simulink model "FusionMODEL_version4"  (R2018a)
settings: Solver=FixedStepAuto  StartTime=0.0  StopTime=SimulationTime  FixedStep=SamplingTime  RelTol=1e-3
values from neighbouring files (symbols this model uses):
  ValidateGRID = true    [SensorFusion_Script0_main.m]
  ValidateLAYOUT = true    [SensorFusion_Script0_main.m]
  VisualizeCLUSTERING = true    [SensorFusion_Script0_main.m]
undefined symbols (not defined in the file or in its folder): ACTIVATE_CAM, ACTIVATE_RAD, CAM1_detTimeStamp, CAM1_MeasNoise, CAM1_objClassID, CAM1_PX, CAM1_PY, CAM1_VX, CAM1_VY, CAM2_detTimeStamp, CAM2_MeasNoise, CAM2_objClassID, CAM2_PX, CAM2_PY, CAM2_VX, CAM2_VY, CAM3_detTimeStamp, CAM3_MeasNoise, CAM3_objClassID, CAM3_PX, CAM3_PY, CAM3_VX, CAM3_VY, CAM4_detTimeStamp, CAM4_MeasNoise, CAM4_objClassID, CAM4_PX, CAM4_PY, CAM4_VX, CAM4_VY, CAM5_detTimeStamp, CAM5_MeasNoise, CAM5_objClassID, CAM5_PX, CAM5_PY, CAM5_VX, CAM5_VY, CAM6_detTimeStamp, CAM6_MeasNoise, CAM6_objClassID, CAM6_PX, CAM6_PY, CAM6_VX, CAM6_VY, CAM7_detTimeStamp, CAM7_MeasNoise, CAM7_objClassID, CAM7_PX, CAM7_PY, CAM7_VX, CAM7_VY, CAM8_detTimeStamp, CAM8_MeasNoise, CAM8_objClassID, CAM8_PX, CAM8_PY, CAM8_VX, CAM8_VY, CAM_nMeas, CAM_TYPE ... (+171)
libraries: simulink_extras x4
(part 8 of 9)

== system FusionMODEL_version4/OBJECT_TRACKER_SENSOR_FUSION/NEAREST_NEIGHBOUR_FOR_CAMERA_MEASUREMENT_GROUPING/NN_MEASUREMENT_GROUPING_WITHIN_EPS/For Iterator Subsystem/NN/PERFORM_NN_CLUSTERING/CHECK_CONDITION ==
  MEAS : Inport
  idx_i : Inport  Port=2
  idx_j : Inport  Port=3
  CLSTR_DATA_INIT : Inport  Port=4
  CLSTR_DATA_PREV : Inport  Port=5
  Bus Selector : BusSelector  OutputSignals=isMeasVisitedFlag
  Bus Selector1 : BusSelector  OutputSignals=MeasArray
  Constant2 : Constant  Value=nn_eps
  LessThanOrEqual1 : RelationalOperator  Operator=<=  OutDataTypeStr=boolean  RndMeth=Simplest
  Logical Operator : Logic  AllPortsSameDT=off  OutDataTypeStr=boolean
  Logical Operator1 : Logic  Operator=NOT  AllPortsSameDT=off  OutDataTypeStr=boolean
  Selector1 : Selector  NumberOfDimensions=2  InputPortWidth=3  IndexOptions=Select all,Index vector (port)  Indices=[1 3],1  OutputSizes=1,1
  Selector2 : Selector  NumberOfDimensions=2  InputPortWidth=3  IndexOptions=Select all,Index vector (port)  Indices=[1 3],1  OutputSizes=1,1
  Selector3 : Selector  NumberOfDimensions=2  InputPortWidth=3  IndexOptions=Select all,Index vector (port)  Indices=[1 3],1  OutputSizes=1,1
  Sqrt : Sqrt  SaturateOnIntegerOverflow=on
  Square : Math  Operator=square  SaturateOnIntegerOverflow=on
  Subtract : Sum  Inputs=+-
  Sum of Elements : Sum  Inputs=+
  Switch6 : Switch  Criteria=u2 > Threshold  Threshold=int32(1)
  Unit Delay : UnitDelay  InitialCondition=CLSTR_SNSR_DELAY_INIT  SampleTime=-1
  isMember : Outport
  CLSTR_DATA : Outport  Port=2
  wires:
  LessThanOrEqual1/1 -> Logical Operator/1
  Bus Selector/1 -> Selector1/1  "<isMeasVisitedFlag>"
  Logical Operator1/1 -> Logical Operator/2
  [x_i] -> Selector2/2
  Bus Selector1/1 -> Selector2/1, Selector3/1  "<MeasArray>"
  Sqrt/1 -> LessThanOrEqual1/1
  idx_i/1 -> [x_i]
  Selector1/1 -> Logical Operator1/1
  idx_j/1 -> [y_j]
  [y_j] -> Selector3/2
  Selector3/1 -> Subtract/2
  Constant2/1 -> LessThanOrEqual1/2
  Selector2/1 -> Subtract/1
  Logical Operator/1 -> isMember/1
  [y_j] -> Selector1/2
  Subtract/1 -> Square/1
  MEAS/1 -> Bus Selector1/1
  Square/1 -> Sum of Elements/1
  Sum of Elements/1 -> Sqrt/1
  [y_j] -> Switch6/2
  CLSTR_DATA_INIT/1 -> Switch6/3
  Switch6/1 -> Bus Selector/1, CLSTR_DATA/1
  CLSTR_DATA_PREV/1 -> Unit Delay/1
  Unit Delay/1 -> Switch6/1

== system FusionMODEL_version4/OBJECT_TRACKER_SENSOR_FUSION/NEAREST_NEIGHBOUR_FOR_CAMERA_MEASUREMENT_GROUPING/NN_MEASUREMENT_GROUPING_WITHIN_EPS/For Iterator Subsystem/NN/PERFORM_NN_CLUSTERING/SET_DATA ==
  isClusterMember : Inport
  CLSTR_DATA : Inport  Port=2
  idx_j : Inport  Port=3
  GET_DATA_FROM_BUS : Subsystem
  SET_CLUSTER_DATA_TO_BUS : Subsystem
  UPDATE_CLUSTER_DATA1 : Subsystem
  CLSTR_DATA_UPD : Outport
  wires:
  SET_CLUSTER_DATA_TO_BUS/1(CLSTR_DATA_UPD) -> CLSTR_DATA_UPD/1
  isClusterMember/1 -> UPDATE_CLUSTER_DATA1/1(FLAG)
  idx_j/1 -> UPDATE_CLUSTER_DATA1/2(idx_j)
  GET_DATA_FROM_BUS/1(<ClusterSizes>) -> UPDATE_CLUSTER_DATA1/3(ClusterSizes)
  GET_DATA_FROM_BUS/2(<ClusterToMeasAssignment>) -> UPDATE_CLUSTER_DATA1/4(Clstr2MeasAssign)
  GET_DATA_FROM_BUS/3(<isMeasVisitedFlag>) -> UPDATE_CLUSTER_DATA1/5(MeasIsVisited)
  GET_DATA_FROM_BUS/4(<nClusters>) -> UPDATE_CLUSTER_DATA1/6(nClusters)
  GET_DATA_FROM_BUS/5(<ClusterMember>) -> UPDATE_CLUSTER_DATA1/7(ClstrMem)
  CLSTR_DATA/1 -> SET_CLUSTER_DATA_TO_BUS/5(CLSTR_DATA), GET_DATA_FROM_BUS/1(CLSTR_DATA)
  UPDATE_CLUSTER_DATA1/1(isVisited) -> SET_CLUSTER_DATA_TO_BUS/1(isMeasVisitedFlag)
  UPDATE_CLUSTER_DATA1/2(ClstrSize) -> SET_CLUSTER_DATA_TO_BUS/2(ClusterSizes)
  UPDATE_CLUSTER_DATA1/3(ClstrAssignment) -> SET_CLUSTER_DATA_TO_BUS/3(ClusterToMeasAssignment)
  UPDATE_CLUSTER_DATA1/4(ClstrMember) -> SET_CLUSTER_DATA_TO_BUS/4(ClusterMember)

== system FusionMODEL_version4/OBJECT_TRACKER_SENSOR_FUSION/SENSOR_LAYOUT_AND_CHRACTERIZATION/PRE_COMPUTE_SENSOR_FOV_GRID/COMPUTE_CAMERA_SNSR_GRID/ComputeCoverageANDConfidence/Compute_Cell_X_and_Y_index/Compute_Cell_X_Y_Center_Coordinate ==
  Cell_id : Inport
  xRes : Inport  Port=2
  xRear : Inport  Port=3
  Cy : Inport  Port=4
  yRes : Inport  Port=5
  yLeft : Inport  Port=6
  Add : Sum  Inputs=+++
  Add1 : Sum  Inputs=+++
  Constant : Constant  Value=single(0.5)
  Divide : Product  Inputs=*/
  Divide1 : Product  Inputs=/*
  Divide2 : Product  Inputs=*/
  Floor : Rounding
  Floor1 : Rounding
  Floor2 : Rounding
  Multiply : Product
  Multiply1 : Product
  Multiply2 : Product
  Subtract : Sum  Inputs=+-
  CellCenterCoordX : Outport
  CellCenterCoordY : Outport  Port=2
  wires:
  Cell_id/1 -> Subtract/1, Divide/1
  Cy/1 -> Multiply/2, Divide/2
  Divide/1 -> Floor/1
  Floor/1 -> [Grid_x_index], Multiply/1
  Multiply/1 -> Subtract/2
  yLeft/1 -> Divide2/1
  yRes/1 -> Multiply1/2, Divide2/2
  Divide1/1 -> Floor1/1
  Divide2/1 -> Floor2/1
  Subtract/1 -> [Grid_y_index]
  Floor1/1 -> Add/2
  [Grid_x_index] -> Add/1
  Constant/1 -> Add1/1, Add/3
  Floor2/1 -> Add1/2
  [Grid_y_index] -> Add1/3
  Add1/1 -> Multiply1/1
  Multiply1/1 -> CellCenterCoordY/1
  xRear/1 -> Divide1/2
  xRes/1 -> Multiply2/1, Divide1/1
  Add/1 -> Multiply2/2
  Multiply2/1 -> CellCenterCoordX/1

== system FusionMODEL_version4/OBJECT_TRACKER_SENSOR_FUSION/SENSOR_LAYOUT_AND_CHRACTERIZATION/PRE_COMPUTE_SENSOR_FOV_GRID/COMPUTE_CAMERA_SNSR_GRID/ComputeCoverageANDConfidence/Compute_Cell_X_and_Y_index/Compute_FOV_Overlap_with_Cell_and_Region_Confidence ==
  Cell_xSnsrCoord : Inport
  Cell_ySnsrCoord : Inport  Port=2
  SnsrIntrinsic : Inport  Port=3
  If : If  ElseIfExpressions=u1 <= 0  ShowElse=off
  If Action Subsystem : Subsystem  TreatAsAtomicUnit=on
  If Action Subsystem2 : Subsystem  TreatAsAtomicUnit=on
  Merge : Merge
  Merge1 : Merge
  RegionConfidence : Outport
  FOVOverlap : Outport  Port=2
  wires:
  If/1 -> If Action Subsystem/Action
  If/2 -> If Action Subsystem2/Action
  If Action Subsystem/1(RegionConfidence) -> [Confi1]
  If Action Subsystem2/1(RegionConfidence) -> [Confi2]
  [Confi1] -> Merge/1
  [Confi2] -> Merge/2
  If Action Subsystem/2(fovOverlap) -> [Overlap1]
  If Action Subsystem2/2(fovOverlap) -> [Overlap2]
  [Overlap1] -> Merge1/1
  [Overlap2] -> Merge1/2
  Cell_xSnsrCoord/1 -> [Cell_xCoord]
  Cell_ySnsrCoord/1 -> [Cell_yCoord]
  [Cell_xCoord] -> If/1
  [Cell_yCoord] -> If Action Subsystem/2(Cell_ySnsrCoord)
  [Cell_xCoord] -> If Action Subsystem/1(Cell_xSnsrCoord)
  SnsrIntrinsic/1 -> [SnsrIntrinsic]
  [SnsrIntrinsic] -> If Action Subsystem/3(SnsrIntrinsic)
  Merge1/1 -> FOVOverlap/1
  Merge/1 -> RegionConfidence/1

== system FusionMODEL_version4/OBJECT_TRACKER_SENSOR_FUSION/SENSOR_LAYOUT_AND_CHRACTERIZATION/PRE_COMPUTE_SENSOR_FOV_GRID/COMPUTE_CAMERA_SNSR_GRID/ComputeCoverageANDConfidence/Compute_Cell_X_and_Y_index/GET_DATA ==
  GridID_vector : Inport
  index : Inport  Port=2
  GridParam : Inport  Port=3
  Bus Selector : BusSelector  OutputSignals=xGridParameters,yGridParameters
  Bus Selector1 : BusSelector  OutputSignals=nGridCellsLat,yRes,yLeft
  Bus Selector2 : BusSelector  OutputSignals=xRes,xRear
  Selector : Selector  NumberOfDimensions=2  InputPortWidth=3  IndexOptions=Select all,Index vector (port)  Indices=[1 3],1  OutputSizes=1,1
  CellID : Outport
  <xRes> : Outport  Port=2
  <xRear> : Outport  Port=3
  <nGridCellsLat> : Outport  Port=4
  <yRes> : Outport  Port=5
  <yLeft> : Outport  Port=6
  wires:
  Bus Selector/2 -> Bus Selector1/1  "<yGridParameters>"
  Bus Selector/1 -> Bus Selector2/1  "<xGridParameters>"
  Bus Selector2/2 -> <xRear>/1  "<xRear>"
  GridParam/1 -> Bus Selector/1
  GridID_vector/1 -> Selector/1
  Selector/1 -> CellID/1
  Bus Selector1/2 -> <yRes>/1  "<yRes>"
  index/1 -> Selector/2
  Bus Selector2/1 -> <xRes>/1  "<xRes>"
  Bus Selector1/1 -> <nGridCellsLat>/1  "<nGridCellsLat>"
  Bus Selector1/3 -> <yLeft>/1  "<yLeft>"

== system FusionMODEL_version4/OBJECT_TRACKER_SENSOR_FUSION/SENSOR_LAYOUT_AND_CHRACTERIZATION/PRE_COMPUTE_SENSOR_FOV_GRID/COMPUTE_CAMERA_SNSR_GRID/ComputeCoverageANDConfidence/Compute_Cell_X_and_Y_index/Transform_Cell_Coordinate_Vehicle_Frame_To_Sensor_Frame ==
  Cell_xCoord : Inport
  Cell_y_Coord : Inport  Port=2
  SensorExtrinsic : Inport  Port=3
  Bus Selector : BusSelector  OutputSignals=RotMat2D,TranslationVec
  Matrix Multiply : Product  Multiplication=Matrix(*)
  Mux : Mux  Inputs=2
  Reshape : Reshape  OutputDimensionality=Column vector (2-D)
  Selector : Selector  NumberOfDimensions=2  InputPortWidth=3  IndexOptions=Index vector (dialog),Select all  Indices=1,1  OutputSizes=1,1
  Selector1 : Selector  NumberOfDimensions=2  InputPortWidth=3  IndexOptions=Index vector (dialog),Select all  Indices=2,1  OutputSizes=1,1
  Subtract : Sum  Inputs=-+
  Transpose : Math  Operator=transpose  SaturateOnIntegerOverflow=on
  Cell_xSnsrCoord : Outport
  Cell_ySnsrCoord : Outport  Port=2
  wires:
  SensorExtrinsic/1 -> Bus Selector/1
  Cell_xCoord/1 -> Mux/1
  Cell_y_Coord/1 -> Mux/2
  Mux/1 -> Reshape/1
  Bus Selector/1 -> Transpose/1  "<RotMat2D>"
  Bus Selector/2 -> Subtract/1  "<TranslationVec>"
  Reshape/1 -> Subtract/2
  Transpose/1 -> Matrix Multiply/1
  Subtract/1 -> Matrix Multiply/2
  Matrix Multiply/1 -> Selector1/1, Selector/1
  Selector/1 -> Cell_xSnsrCoord/1
  Selector1/1 -> Cell_ySnsrCoord/1

== system FusionMODEL_version4/OBJECT_TRACKER_SENSOR_FUSION/SENSOR_LAYOUT_AND_CHRACTERIZATION/PRE_COMPUTE_SENSOR_FOV_GRID/COMPUTE_RADAR_SNSR_GRID/ComputeCoverageANDConfidence/Compute_Cell_X_and_Y_index/Compute_Cell_X_Y_Center_Coordinate ==
  Cell_id : Inport
  xRes : Inport  Port=2
  xRear : Inport  Port=3
  Cy : Inport  Port=4
  yRes : Inport  Port=5
  yLeft : Inport  Port=6
  Add : Sum  Inputs=+++
  Add1 : Sum  Inputs=+++
  Constant : Constant  Value=single(0.5)
  Divide : Product  Inputs=*/
  Divide1 : Product  Inputs=/*
  Divide2 : Product  Inputs=*/
  Floor : Rounding
  Floor1 : Rounding
  Floor2 : Rounding
  Multiply : Product
  Multiply1 : Product
  Multiply2 : Product
  Subtract : Sum  Inputs=+-
  CellCenterCoordX : Outport
  CellCenterCoordY : Outport  Port=2
  wires:
  Cell_id/1 -> Subtract/1, Divide/1
  Cy/1 -> Multiply/2, Divide/2
  Divide/1 -> Floor/1
  Floor/1 -> [Grid_x_index], Multiply/1
  Multiply/1 -> Subtract/2
  yLeft/1 -> Divide2/1
  yRes/1 -> Multiply1/2, Divide2/2
  Divide1/1 -> Floor1/1
  Divide2/1 -> Floor2/1
  Subtract/1 -> [Grid_y_index]
  Floor1/1 -> Add/2
  [Grid_x_index] -> Add/1
  Constant/1 -> Add1/1, Add/3
  Floor2/1 -> Add1/2
  [Grid_y_index] -> Add1/3
  Add1/1 -> Multiply1/1
  Multiply1/1 -> CellCenterCoordY/1
  xRear/1 -> Divide1/2
  xRes/1 -> Multiply2/1, Divide1/1
  Add/1 -> Multiply2/2
  Multiply2/1 -> CellCenterCoordX/1

== system FusionMODEL_version4/OBJECT_TRACKER_SENSOR_FUSION/SENSOR_LAYOUT_AND_CHRACTERIZATION/PRE_COMPUTE_SENSOR_FOV_GRID/COMPUTE_RADAR_SNSR_GRID/ComputeCoverageANDConfidence/Compute_Cell_X_and_Y_index/Compute_FOV_Overlap_with_Cell_and_Region_Confidence ==
  Cell_xSnsrCoord : Inport
  Cell_ySnsrCoord : Inport  Port=2
  SnsrIntrinsic : Inport  Port=3
  If : If  ElseIfExpressions=u1 <= 0  ShowElse=off
  If Action Subsystem : Subsystem  TreatAsAtomicUnit=on
  If Action Subsystem2 : Subsystem  TreatAsAtomicUnit=on
  Merge : Merge
  Merge1 : Merge
  RegionConfidence : Outport
  FOVOverlap : Outport  Port=2
  wires:
  If/1 -> If Action Subsystem/Action
  If/2 -> If Action Subsystem2/Action
  If Action Subsystem/1(RegionConfidence) -> [Confi1]
  If Action Subsystem2/1(RegionConfidence) -> [Confi2]
  [Confi1] -> Merge/1
  [Confi2] -> Merge/2
  If Action Subsystem/2(fovOverlap) -> [Overlap1]
  If Action Subsystem2/2(fovOverlap) -> [Overlap2]
  [Overlap1] -> Merge1/1
  [Overlap2] -> Merge1/2
  Cell_xSnsrCoord/1 -> [Cell_xCoord]
  Cell_ySnsrCoord/1 -> [Cell_yCoord]
  [Cell_xCoord] -> If/1
  [Cell_yCoord] -> If Action Subsystem/2(Cell_ySnsrCoord)
  [Cell_xCoord] -> If Action Subsystem/1(Cell_xSnsrCoord)
  SnsrIntrinsic/1 -> [SnsrIntrinsic]
  [SnsrIntrinsic] -> If Action Subsystem/3(SnsrIntrinsic)
  Merge1/1 -> FOVOverlap/1
  Merge/1 -> RegionConfidence/1

== system FusionMODEL_version4/OBJECT_TRACKER_SENSOR_FUSION/SENSOR_LAYOUT_AND_CHRACTERIZATION/PRE_COMPUTE_SENSOR_FOV_GRID/COMPUTE_RADAR_SNSR_GRID/ComputeCoverageANDConfidence/Compute_Cell_X_and_Y_index/GET_DATA ==
  GridID_vector : Inport
  index : Inport  Port=2
  GridParam : Inport  Port=3
  Bus Selector : BusSelector  OutputSignals=xGridParameters,yGridParameters
  Bus Selector1 : BusSelector  OutputSignals=nGridCellsLat,yRes,yLeft
  Bus Selector2 : BusSelector  OutputSignals=xRes,xRear
  Selector : Selector  NumberOfDimensions=2  InputPortWidth=3  IndexOptions=Select all,Index vector (port)  Indices=[1 3],1  OutputSizes=1,1
  CellID : Outport
  <xRes> : Outport  Port=2
  <xRear> : Outport  Port=3
  <nGridCellsLat> : Outport  Port=4
  <yRes> : Outport  Port=5
  <yLeft> : Outport  Port=6
  wires:
  Bus Selector/2 -> Bus Selector1/1  "<yGridParameters>"
  Bus Selector/1 -> Bus Selector2/1  "<xGridParameters>"
  Bus Selector2/2 -> <xRear>/1  "<xRear>"
  GridParam/1 -> Bus Selector/1
  GridID_vector/1 -> Selector/1
  Selector/1 -> CellID/1
  Bus Selector1/2 -> <yRes>/1  "<yRes>"
  index/1 -> Selector/2
  Bus Selector2/1 -> <xRes>/1  "<xRes>"
  Bus Selector1/1 -> <nGridCellsLat>/1  "<nGridCellsLat>"
  Bus Selector1/3 -> <yLeft>/1  "<yLeft>"

== system FusionMODEL_version4/OBJECT_TRACKER_SENSOR_FUSION/SENSOR_LAYOUT_AND_CHRACTERIZATION/PRE_COMPUTE_SENSOR_FOV_GRID/COMPUTE_RADAR_SNSR_GRID/ComputeCoverageANDConfidence/Compute_Cell_X_and_Y_index/Transform_Cell_Coordinate_Vehicle_Frame_To_Sensor_Frame ==
  Cell_xCoord : Inport
  Cell_y_Coord : Inport  Port=2
  SensorExtrinsic : Inport  Port=3
  Bus Selector : BusSelector  OutputSignals=RotMat2D,TranslationVec
  Matrix Multiply : Product  Multiplication=Matrix(*)
  Mux : Mux  Inputs=2
  Reshape : Reshape  OutputDimensionality=Column vector (2-D)
  Selector : Selector  NumberOfDimensions=2  InputPortWidth=3  IndexOptions=Index vector (dialog),Select all  Indices=1,1  OutputSizes=1,1
  Selector1 : Selector  NumberOfDimensions=2  InputPortWidth=3  IndexOptions=Index vector (dialog),Select all  Indices=2,1  OutputSizes=1,1
  Subtract : Sum  Inputs=-+
  Transpose : Math  Operator=transpose  SaturateOnIntegerOverflow=on
  Cell_xSnsrCoord : Outport
  Cell_ySnsrCoord : Outport  Port=2
  wires:
  SensorExtrinsic/1 -> Bus Selector/1
  Cell_xCoord/1 -> Mux/1
  Cell_y_Coord/1 -> Mux/2
  Mux/1 -> Reshape/1
  Bus Selector/1 -> Transpose/1  "<RotMat2D>"
  Bus Selector/2 -> Subtract/1  "<TranslationVec>"
  Reshape/1 -> Subtract/2
  Transpose/1 -> Matrix Multiply/1
  Subtract/1 -> Matrix Multiply/2
  Matrix Multiply/1 -> Selector1/1, Selector/1
  Selector/1 -> Cell_xSnsrCoord/1
  Selector1/1 -> Cell_ySnsrCoord/1

== system FusionMODEL_version4/OBJECT_TRACKER_SENSOR_FUSION/SENSOR_LAYOUT_AND_CHRACTERIZATION/SET_SENSOR_CALLIBRATION_PARAMETER/SET_CAMERA_SENSOR_PARAM/SET_CAMERA_EXTRINSIC_PARAM/SET_CAMERA_EXTRINSIC_PARAM/CreateRotationMatTranslationVector ==
  yawInstall : Inport
  xMount : Inport  Port=2
  yMount : Inport  Port=3
  Cos : Trigonometry  Operator=cos
  Cos2 : Trigonometry
  Degrees to Radians : simulink_extras/Transformations/Degrees to Radians
  Gain1 : Gain  Gain=-1
  Gain2 : Gain  Gain=ROT_CONVENTION
  Mux : Mux
  Mux1 : Mux  Inputs=2
  Reshape : Reshape  OutputDimensionality=Customize  OutputDimensions=[2 2]
  Reshape1 : Reshape  OutputDimensionality=Column vector (2-D)  OutputDimensions=[2 2]
  RotMatrx : Outport
  TranslationVector : Outport  Port=2
  wires:
  Cos/1 -> [cos_theta], Mux/1
  [cos_theta] -> Mux/4
  Reshape/1 -> RotMatrx/1
  Degrees to Radians/1 -> Cos2/1, Cos/1
  Mux/1 -> Reshape/1
  Cos2/1 -> Mux/2, Gain1/1
  xMount/1 -> Mux1/1
  yMount/1 -> Mux1/2
  Mux1/1 -> Reshape1/1
  Reshape1/1 -> TranslationVector/1
  Gain1/1 -> Mux/3
  yawInstall/1 -> Gain2/1
  Gain2/1 -> Degrees to Radians/1

== system FusionMODEL_version4/OBJECT_TRACKER_SENSOR_FUSION/SENSOR_LAYOUT_AND_CHRACTERIZATION/SET_SENSOR_CALLIBRATION_PARAMETER/SET_RADAR_SENSOR_PARAM/SET_RADAR_EXTRINSIC_PARAM/SET_RADAR_EXTRINSIC_PARAM/CREATE_ROTATION_MATRIX_TRANSLATION_VECTOR ==
  yawInstall : Inport
  xMount : Inport  Port=2
  yMount : Inport  Port=3
  Cos : Trigonometry  Operator=cos
  Cos2 : Trigonometry
  Degrees to Radians : simulink_extras/Transformations/Degrees to Radians
  Gain1 : Gain  Gain=-1
  Gain2 : Gain  Gain=ROT_CONVENTION
  Mux : Mux
  Mux1 : Mux  Inputs=2
  Reshape : Reshape  OutputDimensionality=Customize  OutputDimensions=[2 2]
  Reshape1 : Reshape  OutputDimensionality=Column vector (2-D)  OutputDimensions=[2 2]
  RotMatrx : Outport
  TranslationVector : Outport  Port=2
  wires:
  Cos/1 -> [cos_theta], Mux/1
  [cos_theta] -> Mux/4
  Reshape/1 -> RotMatrx/1
  Degrees to Radians/1 -> Cos2/1, Cos/1
  Mux/1 -> Reshape/1
  Cos2/1 -> Mux/2, Gain1/1
  xMount/1 -> Mux1/1
  yMount/1 -> Mux1/2
  Mux1/1 -> Reshape1/1
  Reshape1/1 -> TranslationVector/1
  Gain1/1 -> Mux/3
  yawInstall/1 -> Gain2/1
  Gain2/1 -> Degrees to Radians/1

== system FusionMODEL_version4/OBJECT_TRACKER_SENSOR_FUSION/SIMPLIFIED_DBSCAN_FOR_RADAR_MEASUREMENT_GROUPING/DBSCAN_MEASUREMENT_GROUPING/FORM_CLUSTER/DBSCAN/DBSCAN_PROPAGATE_AND_EXPAND_CLUSTER/CHECK_CONDITION ==
  memberIdx : Inport
  CLSTR_DATA_INIT : Inport  Port=2
  CLSTR_DATA_PREV : Inport  Port=3
  Bus Selector : BusSelector  OutputSignals=ClusterMember
  Constant : Constant  Value=uint16(0)
  NotEqual : RelationalOperator  Operator=~=  OutDataTypeStr=boolean  RndMeth=Simplest
  Selector : Selector  NumberOfDimensions=2  InputPortWidth=3  IndexOptions=Select all,Index vector (port)  Indices=[1 3],1  OutputSizes=1,1
  Switch6 : Switch  Criteria=u2 > Threshold  Threshold=int32(1)
  Unit Delay : UnitDelay  InitialCondition=CLSTR_SNSR_DELAY_INIT  SampleTime=-1
  isMember : Outport
  MeasIndex : Outport  Port=2
  CLSTR_DATA : Outport  Port=3
  wires:
  Switch6/1 -> CLSTR_DATA/1, Bus Selector/1
  Bus Selector/1 -> Selector/1  "<ClusterMember>"
  memberIdx/1 -> [idx_i], Selector/2
  Selector/1 -> MeasIndex/1, NotEqual/1
  Constant/1 -> NotEqual/2
  NotEqual/1 -> isMember/1
  CLSTR_DATA_INIT/1 -> Switch6/3
  [idx_i] -> Switch6/2
  CLSTR_DATA_PREV/1 -> Unit Delay/1
  Unit Delay/1 -> Switch6/1

== system FusionMODEL_version4/OBJECT_TRACKER_SENSOR_FUSION/SIMPLIFIED_DBSCAN_FOR_RADAR_MEASUREMENT_GROUPING/DBSCAN_MEASUREMENT_GROUPING/FORM_CLUSTER/DBSCAN/DBSCAN_PROPAGATE_AND_EXPAND_CLUSTER/DO_NOT_EXPAND_CLUSTER ==
  CLSTR_DATA : Inport
  Action Port : ActionPort  ActionType=then
  CLSTR_DATA_NO_UPD : Outport
  wires:
  CLSTR_DATA/1 -> CLSTR_DATA_NO_UPD/1

== system FusionMODEL_version4/OBJECT_TRACKER_SENSOR_FUSION/SIMPLIFIED_DBSCAN_FOR_RADAR_MEASUREMENT_GROUPING/DBSCAN_MEASUREMENT_GROUPING/FORM_CLUSTER/DBSCAN/DBSCAN_PROPAGATE_AND_EXPAND_CLUSTER/EXPAND_CLUSTER ==
  CLSTR_DATA : Inport
  nMeas : Inport  Port=2
  idx_i : Inport  Port=3
  measArray : Inport  Port=4
  Action Port : ActionPort  ActionType=else
  CLUSTER_EXPANSION : Subsystem  TreatAsAtomicUnit=on
  CLSTR_DATA_UPD : Outport
  wires:
  CLSTR_DATA/1 -> CLUSTER_EXPANSION/3(CLSTR_DATA)
  idx_i/1 -> CLUSTER_EXPANSION/4(idx_i)
  nMeas/1 -> CLUSTER_EXPANSION/1(nMeas)
  measArray/1 -> CLUSTER_EXPANSION/2(measArray)
  CLUSTER_EXPANSION/1(CLSTR_DATA_UPD) -> CLSTR_DATA_UPD/1

== system FusionMODEL_version4/OBJECT_TRACKER_SENSOR_FUSION/SIMPLIFIED_DBSCAN_FOR_RADAR_MEASUREMENT_GROUPING/DBSCAN_MEASUREMENT_GROUPING/FORM_CLUSTER/DBSCAN/DBSCAN_PROPAGATE_AND_EXPAND_CLUSTER/MERGE_SIGNALS ==
  CLSTR_NO_UPD : Inport
  CLSTR_UPD : Inport  Port=2
  Merge1 : Merge
  CLSTR_DATA : Outport
  wires:
  CLSTR_NO_UPD/1 -> Merge1/1
  Merge1/1 -> CLSTR_DATA/1
  CLSTR_UPD/1 -> Merge1/2

== system FusionMODEL_version4/OBJECT_TRACKER_SENSOR_FUSION/SPATIAL_ALLIGNMENT/CAMERA_MEASUREMENTS_SPATIAL_ALLIGNMENT/For Iterator Subsystem/For Iterator Subsystem/CoordinateTransformation1/InfoExtractor ==
  In1 : Inport
  In2 : Inport  Port=2
  Bus Selector : BusSelector  OutputSignals=px,py,vx,vy,NoiseCovarience
  Bus Selector1 : BusSelector  OutputSignals=RotMat2D,TranslationVec
  <px> : Outport
  <py> : Outport  Port=2
  <vx> : Outport  Port=3
  <vy> : Outport  Port=4
  RotMat2D : Outport  Port=5
  TransVec2D : Outport  Port=6
  MeasNoiseCov : Outport  Port=7
  wires:
  Bus Selector/4 -> <vy>/1  "<vy>"
  Bus Selector/2 -> <py>/1  "<py>"
  In1/1 -> Bus Selector/1
  Bus Selector1/1 -> RotMat2D/1  "<RotMat2D>"
  Bus Selector/3 -> <vx>/1  "<vx>"
  Bus Selector1/2 -> TransVec2D/1  "<TranslationVec>"
  Bus Selector/1 -> <px>/1  "<px>"
  In2/1 -> Bus Selector1/1
  Bus Selector/5 -> MeasNoiseCov/1  "<NoiseCovarience>"

== system FusionMODEL_version4/OBJECT_TRACKER_SENSOR_FUSION/SPATIAL_ALLIGNMENT/CAMERA_MEASUREMENTS_SPATIAL_ALLIGNMENT/For Iterator Subsystem/For Iterator Subsystem/CoordinateTransformation1/Meas_Noise_Cov_Transformation ==
  RotMatrix : Inport
  MeasCovarience : Inport  Port=2
  Assignment : Assignment  NumberOfDimensions=2  DiagnosticForDimensions=Warning  IndexOptions=Index vector (dialog),Index vector (dialog)  Indices=[1 2],[1 2]  OutputSizes=1,1
  Assignment1 : Assignment  NumberOfDimensions=2  DiagnosticForDimensions=Warning  IndexOptions=Index vector (dialog),Index vector (dialog)  Indices=[3 4],[3 4]  OutputSizes=1,1
  Matrix Multiply : Product  Inputs=3  Multiplication=Matrix(*)
  Matrix Multiply1 : Product  Inputs=3  Multiplication=Matrix(*)
  Selector : Selector  NumberOfDimensions=2  InputPortWidth=3  IndexOptions=Index vector (dialog),Index vector (dialog)  Indices=[1 2],[1 2]  OutputSizes=1,1
  Selector1 : Selector  NumberOfDimensions=2  InputPortWidth=3  IndexOptions=Index vector (dialog),Index vector (dialog)  Indices=[3 4],[3 4]  OutputSizes=1,1
  Transpose : Math  Operator=transpose  SaturateOnIntegerOverflow=on
  Transpose1 : Math  Operator=transpose  SaturateOnIntegerOverflow=on
  MeasCovTransformed : Outport
  wires:
  Matrix Multiply/1 -> Assignment/2
  [RotationMat] -> Transpose1/1
  Matrix Multiply1/1 -> Assignment1/2
  RotMatrix/1 -> [RotationMat], Matrix Multiply/1
  [NoiseCov] -> Assignment/1
  Transpose1/1 -> Matrix Multiply1/3
  Selector1/1 -> Matrix Multiply1/2
  Assignment/1 -> Assignment1/1
  Selector/1 -> Matrix Multiply/2
  [RotationMat] -> Matrix Multiply1/1, Transpose/1
  Transpose/1 -> Matrix Multiply/3
  MeasCovarience/1 -> Selector1/1, [NoiseCov], Selector/1
  Assignment1/1 -> MeasCovTransformed/1

== system FusionMODEL_version4/OBJECT_TRACKER_SENSOR_FUSION/SPATIAL_ALLIGNMENT/CAMERA_MEASUREMENTS_SPATIAL_ALLIGNMENT/For Iterator Subsystem/For Iterator Subsystem/CoordinateTransformation1/Position_Transformation ==
  Px : Inport
  Py : Inport  Port=2
  RotationMat : Inport  Port=3
  TranslationVector : Inport  Port=4
  Add : Sum
  Matrix Multiply : Product  Multiplication=Matrix(*)
  Mux : Mux  Inputs=2
  Reshape : Reshape  OutputDimensionality=Column vector (2-D)
  Selector : Selector  InputPortWidth=2  IndexOptions=Index vector (dialog)  Indices=1  OutputSizes=1
  Selector1 : Selector  InputPortWidth=2  IndexOptions=Index vector (dialog)  Indices=2  OutputSizes=1
  PosXcts : Outport
  PosYcts : Outport  Port=2
  wires:
  Reshape/1 -> Matrix Multiply/2
  Px/1 -> Mux/1
  Py/1 -> Mux/2
  Mux/1 -> Reshape/1
  RotationMat/1 -> Matrix Multiply/1
  Matrix Multiply/1 -> Add/1
  TranslationVector/1 -> Add/2
  Add/1 -> Selector1/1, Selector/1
  Selector/1 -> PosXcts/1
  Selector1/1 -> PosYcts/1

== system FusionMODEL_version4/OBJECT_TRACKER_SENSOR_FUSION/SPATIAL_ALLIGNMENT/CAMERA_MEASUREMENTS_SPATIAL_ALLIGNMENT/For Iterator Subsystem/For Iterator Subsystem/CoordinateTransformation1/Subsystem ==
  pxCTS : Inport
  pyCTS : Inport  Port=2
  vxCTS : Inport  Port=3
  vyCTS : Inport  Port=4
  covCTS : Inport  Port=5
  Bus Creator : BusCreator  Inputs=2
  Mux : Mux  Inputs=2
  Reshape : Reshape  OutputDimensionality=Column vector (2-D)
  Selector : Selector  NumberOfDimensions=2  InputPortWidth=3  IndexOptions=Index vector (dialog),Index vector (dialog)  Indices=1:2,1:2  OutputSizes=1,1
  Terminator : Terminator
  Terminator1 : Terminator
  measUpd : Outport
  wires:
  covCTS/1 -> Selector/1
  Bus Creator/1 -> measUpd/1
  pyCTS/1 -> Mux/2
  pxCTS/1 -> Mux/1
  Mux/1 -> Reshape/1
  Reshape/1 -> Bus Creator/1  "stateCTS"
  Selector/1 -> Bus Creator/2  "covCTS"
  vxCTS/1 -> Terminator/1
  vyCTS/1 -> Terminator1/1

== system FusionMODEL_version4/OBJECT_TRACKER_SENSOR_FUSION/SPATIAL_ALLIGNMENT/CAMERA_MEASUREMENTS_SPATIAL_ALLIGNMENT/For Iterator Subsystem/For Iterator Subsystem/CoordinateTransformation1/Velocity_Transformation ==
  Vx : Inport
  Vy : Inport  Port=2
  RotMatrix2D : Inport  Port=3
  Matrix Multiply : Product  Multiplication=Matrix(*)
  Mux : Mux  Inputs=2
  Reshape : Reshape  OutputDimensionality=Column vector (2-D)
  Selector : Selector  InputPortWidth=2  IndexOptions=Index vector (dialog)  Indices=1  OutputSizes=1
  Selector1 : Selector  InputPortWidth=2  IndexOptions=Index vector (dialog)  Indices=2  OutputSizes=1
  VelXcts : Outport
  VelYcts : Outport  Port=2
  wires:
  Vy/1 -> Mux/2
  RotMatrix2D/1 -> Matrix Multiply/1
  Vx/1 -> Mux/1
  Mux/1 -> Reshape/1
  Reshape/1 -> Matrix Multiply/2
  Matrix Multiply/1 -> Selector1/1, Selector/1
  Selector/1 -> VelXcts/1
  Selector1/1 -> VelYcts/1

== system FusionMODEL_version4/OBJECT_TRACKER_SENSOR_FUSION/SPATIAL_ALLIGNMENT/RADAR_MEASUREMENTS_SPATIAL_ALLIGNMENT/RADAR_MEASUREMENTS_SPATIAL_ALLIGNMENT/COORDINATE_TRANSFORMATION/COORDINATE_TRANSFORMATION/GET_DATA ==
  In1 : Inport
  In2 : Inport  Port=2
  Bus Selector : BusSelector  OutputSignals=px,py,vx,vy,NoiseCovarience
  Bus Selector1 : BusSelector  OutputSignals=RotMat2D,TranslationVec
  <px> : Outport
  <py> : Outport  Port=2
  <vx> : Outport  Port=3
  <vy> : Outport  Port=4
  RotMat2D : Outport  Port=5
  TransVec2D : Outport  Port=6
  MeasNoiseCov : Outport  Port=7
  wires:
  Bus Selector/4 -> <vy>/1  "<vy>"
  Bus Selector/2 -> <py>/1  "<py>"
  In1/1 -> Bus Selector/1
  Bus Selector1/1 -> RotMat2D/1  "<RotMat2D>"
  Bus Selector/3 -> <vx>/1  "<vx>"
  Bus Selector1/2 -> TransVec2D/1  "<TranslationVec>"
  Bus Selector/1 -> <px>/1  "<px>"
  In2/1 -> Bus Selector1/1
  Bus Selector/5 -> MeasNoiseCov/1  "<NoiseCovarience>"

== system FusionMODEL_version4/OBJECT_TRACKER_SENSOR_FUSION/SPATIAL_ALLIGNMENT/RADAR_MEASUREMENTS_SPATIAL_ALLIGNMENT/RADAR_MEASUREMENTS_SPATIAL_ALLIGNMENT/COORDINATE_TRANSFORMATION/COORDINATE_TRANSFORMATION/MEAS_NOISE_COV_TRANSFORMATION ==
  RotMatrix : Inport
  MeasCovarience : Inport  Port=2
  Assignment : Assignment  NumberOfDimensions=2  DiagnosticForDimensions=Warning  IndexOptions=Index vector (dialog),Index vector (dialog)  Indices=[1 2],[1 2]  OutputSizes=1,1
  Assignment1 : Assignment  NumberOfDimensions=2  DiagnosticForDimensions=Warning  IndexOptions=Index vector (dialog),Index vector (dialog)  Indices=[3 4],[3 4]  OutputSizes=1,1
  Matrix Multiply : Product  Inputs=3  Multiplication=Matrix(*)
  Matrix Multiply1 : Product  Inputs=3  Multiplication=Matrix(*)
  Selector : Selector  NumberOfDimensions=2  InputPortWidth=3  IndexOptions=Index vector (dialog),Index vector (dialog)  Indices=[1 2],[1 2]  OutputSizes=1,1
  Selector1 : Selector  NumberOfDimensions=2  InputPortWidth=3  IndexOptions=Index vector (dialog),Index vector (dialog)  Indices=[3 4],[3 4]  OutputSizes=1,1
  Transpose : Math  Operator=transpose  SaturateOnIntegerOverflow=on
  Transpose1 : Math  Operator=transpose  SaturateOnIntegerOverflow=on
  MeasCovTransformed : Outport
  wires:
  Matrix Multiply/1 -> Assignment/2
  [RotationMat] -> Transpose1/1
  Matrix Multiply1/1 -> Assignment1/2
  RotMatrix/1 -> [RotationMat], Matrix Multiply/1
  [NoiseCov] -> Assignment/1
  Transpose1/1 -> Matrix Multiply1/3
  Selector1/1 -> Matrix Multiply1/2
  Assignment/1 -> Assignment1/1
  Selector/1 -> Matrix Multiply/2
  [RotationMat] -> Matrix Multiply1/1, Transpose/1
  Transpose/1 -> Matrix Multiply/3
  MeasCovarience/1 -> Selector1/1, [NoiseCov], Selector/1
  Assignment1/1 -> MeasCovTransformed/1

== system FusionMODEL_version4/OBJECT_TRACKER_SENSOR_FUSION/SPATIAL_ALLIGNMENT/RADAR_MEASUREMENTS_SPATIAL_ALLIGNMENT/RADAR_MEASUREMENTS_SPATIAL_ALLIGNMENT/COORDINATE_TRANSFORMATION/COORDINATE_TRANSFORMATION/POSITION_TRANSFORMATION ==
  Px : Inport
  Py : Inport  Port=2
  RotationMat : Inport  Port=3
  TranslationVector : Inport  Port=4
  Add : Sum
  Matrix Multiply : Product  Multiplication=Matrix(*)
  Mux : Mux  Inputs=2
  Reshape : Reshape  OutputDimensionality=Column vector (2-D)
  Selector : Selector  InputPortWidth=2  IndexOptions=Index vector (dialog)  Indices=1  OutputSizes=1
  Selector1 : Selector  InputPortWidth=2  IndexOptions=Index vector (dialog)  Indices=2  OutputSizes=1
  PosXcts : Outport
  PosYcts : Outport  Port=2
  wires:
  Reshape/1 -> Matrix Multiply/2
  Px/1 -> Mux/1
  Py/1 -> Mux/2
  Mux/1 -> Reshape/1
  RotationMat/1 -> Matrix Multiply/1
  Matrix Multiply/1 -> Add/1
  TranslationVector/1 -> Add/2
  Add/1 -> Selector1/1, Selector/1
  Selector/1 -> PosXcts/1
  Selector1/1 -> PosYcts/1

== system FusionMODEL_version4/OBJECT_TRACKER_SENSOR_FUSION/SPATIAL_ALLIGNMENT/RADAR_MEASUREMENTS_SPATIAL_ALLIGNMENT/RADAR_MEASUREMENTS_SPATIAL_ALLIGNMENT/COORDINATE_TRANSFORMATION/COORDINATE_TRANSFORMATION/SET_DATA ==
  pxCTS : Inport
  pyCTS : Inport  Port=2
  vxCTS : Inport  Port=3
  vyCTS : Inport  Port=4
  covCTS : Inport  Port=5
  Bus Creator : BusCreator  Inputs=2
  Mux : Mux  Inputs=2
  Reshape : Reshape  OutputDimensionality=Column vector (2-D)
  Selector : Selector  NumberOfDimensions=2  InputPortWidth=3  IndexOptions=Index vector (dialog),Index vector (dialog)  Indices=1:2,1:2  OutputSizes=1,1
  Terminator : Terminator
  Terminator1 : Terminator
  measUpd : Outport
  wires:
  covCTS/1 -> Selector/1
  Bus Creator/1 -> measUpd/1
  pyCTS/1 -> Mux/2
  pxCTS/1 -> Mux/1
  Mux/1 -> Reshape/1
  Reshape/1 -> Bus Creator/1  "stateCTS"
  Selector/1 -> Bus Creator/2  "covCTS"
  vxCTS/1 -> Terminator/1
  vyCTS/1 -> Terminator1/1

== system FusionMODEL_version4/OBJECT_TRACKER_SENSOR_FUSION/SPATIAL_ALLIGNMENT/RADAR_MEASUREMENTS_SPATIAL_ALLIGNMENT/RADAR_MEASUREMENTS_SPATIAL_ALLIGNMENT/COORDINATE_TRANSFORMATION/COORDINATE_TRANSFORMATION/VELOCITY_TRANSFORMATION ==
  Vx : Inport
  Vy : Inport  Port=2
  RotMatrix2D : Inport  Port=3
  Matrix Multiply : Product  Multiplication=Matrix(*)
  Mux : Mux  Inputs=2
  Reshape : Reshape  OutputDimensionality=Column vector (2-D)
  Selector : Selector  InputPortWidth=2  IndexOptions=Index vector (dialog)  Indices=1  OutputSizes=1
  Selector1 : Selector  InputPortWidth=2  IndexOptions=Index vector (dialog)  Indices=2  OutputSizes=1
  VelXcts : Outport
  VelYcts : Outport  Port=2
  wires:
  Vy/1 -> Mux/2
  RotMatrix2D/1 -> Matrix Multiply/1
  Vx/1 -> Mux/1
  Mux/1 -> Reshape/1
  Reshape/1 -> Matrix Multiply/2
  Matrix Multiply/1 -> Selector1/1, Selector/1
  Selector/1 -> VelXcts/1
  Selector1/1 -> VelYcts/1

== system FusionMODEL_version4/OBJECT_TRACKER_SENSOR_FUSION/NEAREST_NEIGHBOUR_FOR_CAMERA_MEASUREMENT_GROUPING/NN_MEASUREMENT_GROUPING_WITHIN_EPS/For Iterator Subsystem/NN/PERFORM_NN_CLUSTERING/SET_DATA/GET_DATA_FROM_BUS ==
  CLSTR_DATA : Inport
  Bus Selector : BusSelector  OutputSignals=ClusterSizes,ClusterToMeasAssignment,isMeasVisitedFlag,nClusters,ClusterMember
  <ClusterSizes> : Outport
  <ClusterToMeasAssignment> : Outport  Port=2
  <isMeasVisitedFlag> : Outport  Port=3
  <nClusters> : Outport  Port=4
  <ClusterMember> : Outport  Port=5
  wires:
  CLSTR_DATA/1 -> Bus Selector/1
  Bus Selector/2 -> <ClusterToMeasAssignment>/1  "<ClusterToMeasAssignment>"
  Bus Selector/3 -> <isMeasVisitedFlag>/1  "<isMeasVisitedFlag>"
  Bus Selector/5 -> <ClusterMember>/1  "<ClusterMember>"
  Bus Selector/1 -> <ClusterSizes>/1  "<ClusterSizes>"
  Bus Selector/4 -> <nClusters>/1  "<nClusters>"

== system FusionMODEL_version4/OBJECT_TRACKER_SENSOR_FUSION/NEAREST_NEIGHBOUR_FOR_CAMERA_MEASUREMENT_GROUPING/NN_MEASUREMENT_GROUPING_WITHIN_EPS/For Iterator Subsystem/NN/PERFORM_NN_CLUSTERING/SET_DATA/SET_CLUSTER_DATA_TO_BUS ==
  isMeasVisitedFlag : Inport
  ClusterSizes : Inport  Port=2
  ClusterToMeasAssignment : Inport  Port=3
  ClusterMember : Inport  Port=4
  CLSTR_DATA : Inport  Port=5
  Bus Creator : BusCreator  Inputs=7  OutDataTypeStr=Bus: CLUSTER_DATA_STRUCT_SNSR  NonVirtualBus=on
      settings: InheritFromInputs=off
  Bus Selector1 : BusSelector  OutputSignals=ClusterCenter,ClusterCovariance,ClusterSizes,ClusterToMeasAssignment,isMeasVisitedFlag,nClusters,ClusterMember
  Terminator{,1..2,4} (4 alike) : Terminator
  CLSTR_DATA_UPD : Outport
  wires:
  Bus Selector1/6 -> Bus Creator/6  "<nClusters>"
  Bus Selector1/1 -> Bus Creator/1  "<ClusterCenter>"
  Bus Selector1/2 -> Bus Creator/2  "<ClusterCovariance>"
  Bus Selector1/4 -> Terminator2/1  "<ClusterToMeasAssignment>"
  Bus Selector1/7 -> Terminator4/1  "<ClusterMember>"
  Bus Selector1/5 -> Terminator/1  "<isMeasVisitedFlag>"
  Bus Selector1/3 -> Terminator1/1  "<ClusterSizes>"
  CLSTR_DATA/1 -> Bus Selector1/1
  Bus Creator/1 -> CLSTR_DATA_UPD/1
  ClusterToMeasAssignment/1 -> Bus Creator/4  "ClusterToMeasAssignment"
  isMeasVisitedFlag/1 -> Bus Creator/5  "isMeasVisitedFlag"
  ClusterMember/1 -> Bus Creator/7  "ClusterMember"
  ClusterSizes/1 -> Bus Creator/3  "ClusterSizes"

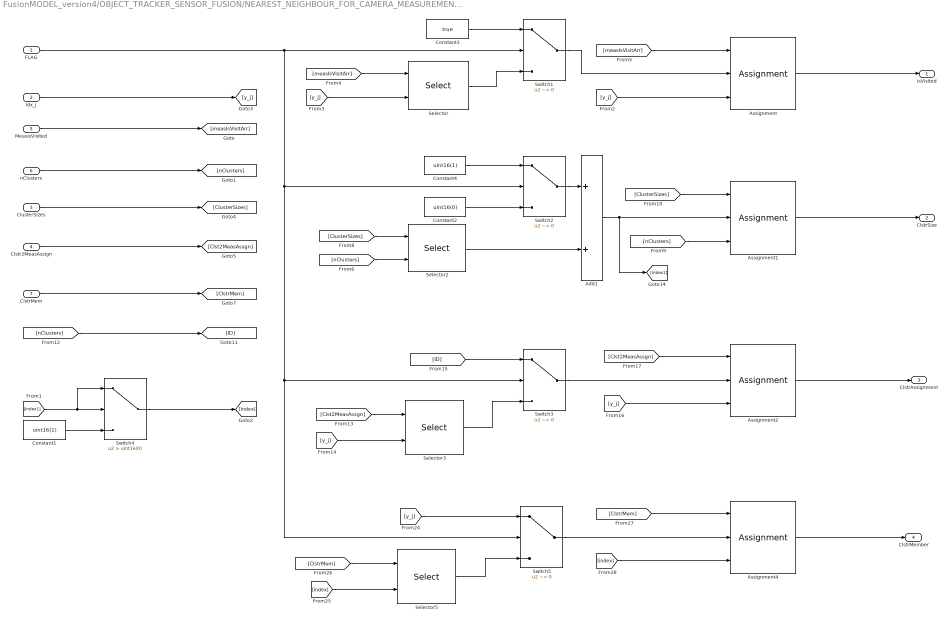
== system FusionMODEL_version4/OBJECT_TRACKER_SENSOR_FUSION/NEAREST_NEIGHBOUR_FOR_CAMERA_MEASUREMENT_GROUPING/NN_MEASUREMENT_GROUPING_WITHIN_EPS/For Iterator Subsystem/NN/PERFORM_NN_CLUSTERING/SET_DATA/UPDATE_CLUSTER_DATA1 ==
  FLAG : Inport
  idx_j : Inport  Port=2
  ClusterSizes : Inport  Port=3
  Clstr2MeasAssign : Inport  Port=4
  MeasIsVisited : Inport  Port=5
  nClusters : Inport  Port=6
  ClstrMem : Inport  Port=7
  Add1 : Sum
  Assignment{,1..2,4} (4 alike) : Assignment  NumberOfDimensions=2  DiagnosticForDimensions=Warning  IndexOptions=Assign all,Index vector (port)  Indices=1,1  OutputSizes=1,1
  Constant1 : Constant  Value=uint16(1)
  Constant2 : Constant  Value=uint16(0)
  Constant3 : Constant  Value=true
  Constant4 : Constant  Value=uint16(1)
  Selector{,2..3,5} (4 alike) : Selector  NumberOfDimensions=2  InputPortWidth=3  IndexOptions=Select all,Index vector (port)  Indices=[1 3],1  OutputSizes=1,1
  Switch{1..3,5} (4 alike) : Switch  Criteria=u2 ~= 0
  Switch4 : Switch  Criteria=u2 > Threshold  Threshold=uint16(0)
  isVisited : Outport
  ClstrSize : Outport  Port=2
  ClstrAssignment : Outport  Port=3
  ClstrMember : Outport  Port=4
  wires:
  [ClusterSizes] -> Assignment1/1
  [y_j] -> Selector3/2
  Switch1/1 -> Assignment/2
  [y_j] -> Assignment/3
  [ID] -> Switch3/1
  FLAG/1 -> Switch1/2, Switch5/2, Switch3/2, Switch2/2
  Assignment4/1 -> ClstrMember/1
  Selector3/1 -> Switch3/3
  Selector/1 -> Switch1/3
  [ClusterSizes] -> Selector2/1
  [Clst2MeasAssgn] -> Assignment2/1
  Constant3/1 -> Switch1/1
  Assignment/1 -> isVisited/1
  Switch5/1 -> Assignment4/2
  [ClstrMem] -> Selector5/1
  [measIsVisitArr] -> Assignment/1
  [y_j] -> Selector/2
  [y_j] -> Switch5/1
  [measIsVisitArr] -> Selector/1
  [nClusters] -> [ID]
  Add1/1 -> Assignment1/2, [index1]
  [nClusters] -> Assignment1/3
  Constant4/1 -> Switch2/1
  Constant2/1 -> Switch2/3
  [index] -> Assignment4/3
  [ClstrMem] -> Assignment4/1
  Assignment1/1 -> ClstrSize/1
  Selector5/1 -> Switch5/3
  Switch3/1 -> Assignment2/2
  Selector2/1 -> Add1/2
  [Clst2MeasAssgn] -> Selector3/1
  Switch2/1 -> Add1/1
  Assignment2/1 -> ClstrAssignment/1
  [index] -> Selector5/2
  [nClusters] -> Selector2/2
  [y_j] -> Assignment2/3
  idx_j/1 -> [y_j]
  MeasIsVisited/1 -> [measIsVisitArr]
  nClusters/1 -> [nClusters]
  ClusterSizes/1 -> [ClusterSizes]
  Clstr2MeasAssign/1 -> [Clst2MeasAssgn]
  ClstrMem/1 -> [ClstrMem]
  [index1] -> Switch4/1, Switch4/2
  Constant1/1 -> Switch4/3
  Switch4/1 -> [index]

== system FusionMODEL_version4/OBJECT_TRACKER_SENSOR_FUSION/SENSOR_LAYOUT_AND_CHRACTERIZATION/PRE_COMPUTE_SENSOR_FOV_GRID/COMPUTE_CAMERA_SNSR_GRID/ComputeCoverageANDConfidence/Compute_Cell_X_and_Y_index/Compute_FOV_Overlap_with_Cell_and_Region_Confidence/If Action Subsystem ==
  Cell_xSnsrCoord : Inport
  Cell_ySnsrCoord : Inport  Port=2
  SnsrIntrinsic : Inport  Port=3
  Action Port : ActionPort  ActionType=then
  Check_IF_Within_FOV : Subsystem
  Compute_Range_Azimuth : Subsystem
  If : If  IfExpression=u1==1
  If Action Subsystem1 : Subsystem  TreatAsAtomicUnit=on
  If Action Subsystem2 : Subsystem  TreatAsAtomicUnit=on
  Merge : Merge
  Merge1 : Merge
  RegionConfidence : Outport
  fovOverlap : Outport  Port=2
  wires:
  Cell_xSnsrCoord/1 -> [x], Compute_Range_Azimuth/1(x)
  Cell_ySnsrCoord/1 -> [y], Compute_Range_Azimuth/2(y)
  Compute_Range_Azimuth/1(Range) -> Check_IF_Within_FOV/1(Range)
  Compute_Range_Azimuth/2(Azimuth) -> Check_IF_Within_FOV/2(In2)
  SnsrIntrinsic/1 -> Check_IF_Within_FOV/3(SnsrIntrinsic)
  Check_IF_Within_FOV/1(isWithinFOV) -> [FLAG]
  [FLAG] -> If/1
  If/2 -> If Action Subsystem2/Action
  If/1 -> If Action Subsystem1/Action
  [Overlap1] -> Merge1/1
  [Confi2] -> Merge/2
  [Overlap2] -> Merge1/2
  [Confi1] -> Merge/1
  If Action Subsystem1/1(RangeConfidence) -> [Confi1]
  If Action Subsystem2/1(RegionConfidence) -> [Confi2]
  If Action Subsystem1/2(fovOverlap) -> [Overlap1]
  If Action Subsystem2/2(fovOverlap) -> [Overlap2]
  Merge/1 -> RegionConfidence/1
  Merge1/1 -> fovOverlap/1
  [y] -> If Action Subsystem1/2(y)
  [x] -> If Action Subsystem1/1(x)

== system FusionMODEL_version4/OBJECT_TRACKER_SENSOR_FUSION/SENSOR_LAYOUT_AND_CHRACTERIZATION/PRE_COMPUTE_SENSOR_FOV_GRID/COMPUTE_CAMERA_SNSR_GRID/ComputeCoverageANDConfidence/Compute_Cell_X_and_Y_index/Compute_FOV_Overlap_with_Cell_and_Region_Confidence/If Action Subsystem2 ==
  Action Port : ActionPort  ActionType=elseif
  Constant : Constant  Value=single(0)
  Constant1 : Constant  Value=false
  RegionConfidence : Outport
  fovOverlap : Outport  Port=2
  wires:
  Constant/1 -> RegionConfidence/1
  Constant1/1 -> fovOverlap/1

== system FusionMODEL_version4/OBJECT_TRACKER_SENSOR_FUSION/SENSOR_LAYOUT_AND_CHRACTERIZATION/PRE_COMPUTE_SENSOR_FOV_GRID/COMPUTE_RADAR_SNSR_GRID/ComputeCoverageANDConfidence/Compute_Cell_X_and_Y_index/Compute_FOV_Overlap_with_Cell_and_Region_Confidence/If Action Subsystem ==
  Cell_xSnsrCoord : Inport
  Cell_ySnsrCoord : Inport  Port=2
  SnsrIntrinsic : Inport  Port=3
  Action Port : ActionPort  ActionType=then
  Check_IF_Within_FOV : Subsystem
  Compute_Range_Azimuth : Subsystem
  If : If  IfExpression=u1==1
  If Action Subsystem1 : Subsystem  TreatAsAtomicUnit=on
  If Action Subsystem2 : Subsystem  TreatAsAtomicUnit=on
  Merge : Merge
  Merge1 : Merge
  RegionConfidence : Outport
  fovOverlap : Outport  Port=2
  wires:
  Cell_xSnsrCoord/1 -> [x], Compute_Range_Azimuth/1(x)
  Cell_ySnsrCoord/1 -> [y], Compute_Range_Azimuth/2(y)
  Compute_Range_Azimuth/1(Range) -> Check_IF_Within_FOV/1(Range)
  Compute_Range_Azimuth/2(Azimuth) -> Check_IF_Within_FOV/2(In2)
  SnsrIntrinsic/1 -> Check_IF_Within_FOV/3(SnsrIntrinsic)
  Check_IF_Within_FOV/1(isWithinFOV) -> [FLAG]
  [FLAG] -> If/1
  If/2 -> If Action Subsystem2/Action
  If/1 -> If Action Subsystem1/Action
  [Overlap1] -> Merge1/1
  [Confi2] -> Merge/2
  [Overlap2] -> Merge1/2
  [Confi1] -> Merge/1
  If Action Subsystem1/1(RangeConfidence) -> [Confi1]
  If Action Subsystem2/1(RegionConfidence) -> [Confi2]
  If Action Subsystem1/2(fovOverlap) -> [Overlap1]
  If Action Subsystem2/2(fovOverlap) -> [Overlap2]
  Merge/1 -> RegionConfidence/1
  Merge1/1 -> fovOverlap/1
  [y] -> If Action Subsystem1/2(y)
  [x] -> If Action Subsystem1/1(x)

== system FusionMODEL_version4/OBJECT_TRACKER_SENSOR_FUSION/SENSOR_LAYOUT_AND_CHRACTERIZATION/PRE_COMPUTE_SENSOR_FOV_GRID/COMPUTE_RADAR_SNSR_GRID/ComputeCoverageANDConfidence/Compute_Cell_X_and_Y_index/Compute_FOV_Overlap_with_Cell_and_Region_Confidence/If Action Subsystem2 ==
  Action Port : ActionPort  ActionType=elseif
  Constant : Constant  Value=single(0)
  Constant1 : Constant  Value=false
  RegionConfidence : Outport
  fovOverlap : Outport  Port=2
  wires:
  Constant/1 -> RegionConfidence/1
  Constant1/1 -> fovOverlap/1

== system FusionMODEL_version4/OBJECT_TRACKER_SENSOR_FUSION/SIMPLIFIED_DBSCAN_FOR_RADAR_MEASUREMENT_GROUPING/DBSCAN_MEASUREMENT_GROUPING/FORM_CLUSTER/DBSCAN/DBSCAN_PROPAGATE_AND_EXPAND_CLUSTER/EXPAND_CLUSTER/CLUSTER_EXPANSION ==
  nMeas : Inport
  measArray : Inport  Port=2
  CLSTR_DATA : Inport  Port=3
  idx_i : Inport  Port=4
  CHECK_CONDITION : Subsystem
  For Iterator : ForIterator  ResetStates=reset  IterationSource=external
  SET_DATA : Subsystem
  CLSTR_DATA_UPD : Outport
  wires:
  CHECK_CONDITION/1(isMember) -> SET_DATA/1(isClusterMember)
  CHECK_CONDITION/2(CLSTR_DATA) -> SET_DATA/2(CLSTR_DATA)
  CLSTR_DATA/1 -> CHECK_CONDITION/4(CLSTR_DATA_INIT)
  [y_j] -> SET_DATA/3(idx_j)
  SET_DATA/1(CLSTR_DATA_UPD) -> CHECK_CONDITION/5(CLSTR_DATA_PREV), CLSTR_DATA_UPD/1
  For Iterator/1 -> [y_j], CHECK_CONDITION/3(idx_j)
  nMeas/1 -> For Iterator/1
  measArray/1 -> CHECK_CONDITION/1(MEAS)
  idx_i/1 -> CHECK_CONDITION/2(idx_i)

== system FusionMODEL_version4/OBJECT_TRACKER_SENSOR_FUSION/SENSOR_LAYOUT_AND_CHRACTERIZATION/PRE_COMPUTE_SENSOR_FOV_GRID/COMPUTE_CAMERA_SNSR_GRID/ComputeCoverageANDConfidence/Compute_Cell_X_and_Y_index/Compute_FOV_Overlap_with_Cell_and_Region_Confidence/If Action Subsystem/Check_IF_Within_FOV ==
  Range : Inport
  In2 : Inport  Port=2
  SnsrIntrinsic : Inport  Port=3
  Abs : Abs
  Bus Selector : BusSelector  OutputSignals=MaxRange,MaxAzimuth
  GreaterThanOrEqual : RelationalOperator  Operator=<=  OutDataTypeStr=boolean  RndMeth=Simplest
  GreaterThanOrEqual1 : RelationalOperator  OutDataTypeStr=boolean  RndMeth=Simplest
  Logical Operator : Logic  AllPortsSameDT=off  OutDataTypeStr=boolean
  isWithinFOV : Outport
  wires:
  Bus Selector/1 -> GreaterThanOrEqual/2  "<MaxRange>"
  Logical Operator/1 -> isWithinFOV/1
  GreaterThanOrEqual/1 -> Logical Operator/1
  SnsrIntrinsic/1 -> Bus Selector/1
  Range/1 -> GreaterThanOrEqual/1
  GreaterThanOrEqual1/1 -> Logical Operator/2
  Bus Selector/2 -> GreaterThanOrEqual1/1  "<MaxAzimuth>"
  In2/1 -> Abs/1
  Abs/1 -> GreaterThanOrEqual1/2

== system FusionMODEL_version4/OBJECT_TRACKER_SENSOR_FUSION/SENSOR_LAYOUT_AND_CHRACTERIZATION/PRE_COMPUTE_SENSOR_FOV_GRID/COMPUTE_CAMERA_SNSR_GRID/ComputeCoverageANDConfidence/Compute_Cell_X_and_Y_index/Compute_FOV_Overlap_with_Cell_and_Region_Confidence/If Action Subsystem/Compute_Range_Azimuth ==
  x : Inport
  y : Inport  Port=2
  Add : Sum
  Atan : Trigonometry  Operator=atan
  Divide : Product  Inputs=*/
  Radians to Degrees : simulink_extras/Transformations/Radians to Degrees
  Sqrt : Sqrt  SaturateOnIntegerOverflow=on
  Square : Math  Operator=square  SaturateOnIntegerOverflow=on
  Square1 : Math  Operator=square  SaturateOnIntegerOverflow=on
  Range : Outport
  Azimuth : Outport  Port=2
  wires:
  Square/1 -> Add/1
  Square1/1 -> Add/2
  Add/1 -> Sqrt/1
  Atan/1 -> Radians to Degrees/1
  Sqrt/1 -> Range/1
  Radians to Degrees/1 -> Azimuth/1
  Divide/1 -> Atan/1
  y/1 -> Square1/1, Divide/1
  x/1 -> Square/1, Divide/2

== system FusionMODEL_version4/OBJECT_TRACKER_SENSOR_FUSION/SENSOR_LAYOUT_AND_CHRACTERIZATION/PRE_COMPUTE_SENSOR_FOV_GRID/COMPUTE_CAMERA_SNSR_GRID/ComputeCoverageANDConfidence/Compute_Cell_X_and_Y_index/Compute_FOV_Overlap_with_Cell_and_Region_Confidence/If Action Subsystem/If Action Subsystem1 ==
  x : Inport
  y : Inport  Port=2
  Action Port : ActionPort  ActionType=then
  If Action Subsystem : Subsystem  TreatAsAtomicUnit=on
  If Action Subsystem1 : Subsystem  TreatAsAtomicUnit=on
  If Action Subsystem2 : Subsystem  TreatAsAtomicUnit=on
  If Action Subsystem3 : Subsystem  TreatAsAtomicUnit=on
  If Action Subsystem4 : Subsystem  TreatAsAtomicUnit=on
  If Action Subsystem5 : Subsystem  TreatAsAtomicUnit=on
  If Action Subsystem6 : Subsystem  TreatAsAtomicUnit=on
  If Action Subsystem7 : Subsystem  TreatAsAtomicUnit=on
  Subsystem2 : Subsystem
  Subsystem3 : Subsystem
  Subsystem4 : Subsystem
  RangeConfidence : Outport
  fovOverlap : Outport  Port=2
  wires:
  y/1 -> Subsystem2/1(y)
  x/1 -> Subsystem3/1(x)
  Subsystem2/1(y1) -> If Action Subsystem4/Action
  Subsystem3/3(x3) -> If Action Subsystem2/Action
  Subsystem3/2(x2) -> If Action Subsystem1/Action
  Subsystem2/3(y3) -> If Action Subsystem6/Action
  Subsystem3/4(x4) -> If Action Subsystem3/Action
  Subsystem2/4(y4) -> If Action Subsystem7/Action
  Subsystem2/2(y2) -> If Action Subsystem5/Action
  Subsystem3/1(x1) -> If Action Subsystem/Action
  If Action Subsystem/1(x1) -> Subsystem4/1(x1)
  If Action Subsystem1/1(x1) -> Subsystem4/2(x2)
  If Action Subsystem2/1(x1) -> Subsystem4/3(x3)
  If Action Subsystem3/1(x1) -> Subsystem4/4(x4)
  If Action Subsystem4/1(x1) -> Subsystem4/5(y1)
  If Action Subsystem5/1(x1) -> Subsystem4/6(y2)
  If Action Subsystem6/1(x1) -> Subsystem4/7(y3)
  If Action Subsystem7/1(x1) -> Subsystem4/8(y4)
  Subsystem4/1(RegionConfidence) -> RangeConfidence/1
  Subsystem4/2(FOVOverlap) -> fovOverlap/1

== system FusionMODEL_version4/OBJECT_TRACKER_SENSOR_FUSION/SENSOR_LAYOUT_AND_CHRACTERIZATION/PRE_COMPUTE_SENSOR_FOV_GRID/COMPUTE_CAMERA_SNSR_GRID/ComputeCoverageANDConfidence/Compute_Cell_X_and_Y_index/Compute_FOV_Overlap_with_Cell_and_Region_Confidence/If Action Subsystem/If Action Subsystem2 ==
  Action Port : ActionPort  ActionType=else
  Constant : Constant  Value=single(0)
  Constant1 : Constant  Value=false
  RegionConfidence : Outport
  fovOverlap : Outport  Port=2
  wires:
  Constant/1 -> RegionConfidence/1
  Constant1/1 -> fovOverlap/1

== system FusionMODEL_version4/OBJECT_TRACKER_SENSOR_FUSION/SENSOR_LAYOUT_AND_CHRACTERIZATION/PRE_COMPUTE_SENSOR_FOV_GRID/COMPUTE_RADAR_SNSR_GRID/ComputeCoverageANDConfidence/Compute_Cell_X_and_Y_index/Compute_FOV_Overlap_with_Cell_and_Region_Confidence/If Action Subsystem/Check_IF_Within_FOV ==
  Range : Inport
  In2 : Inport  Port=2
  SnsrIntrinsic : Inport  Port=3
  Abs : Abs
  Bus Selector : BusSelector  OutputSignals=MaxRange,MaxAzimuth
  GreaterThanOrEqual : RelationalOperator  Operator=<=  OutDataTypeStr=boolean  RndMeth=Simplest
  GreaterThanOrEqual1 : RelationalOperator  OutDataTypeStr=boolean  RndMeth=Simplest
  Logical Operator : Logic  AllPortsSameDT=off  OutDataTypeStr=boolean
  isWithinFOV : Outport
  wires:
  Bus Selector/1 -> GreaterThanOrEqual/2  "<MaxRange>"
  Logical Operator/1 -> isWithinFOV/1
  GreaterThanOrEqual/1 -> Logical Operator/1
  SnsrIntrinsic/1 -> Bus Selector/1
  Range/1 -> GreaterThanOrEqual/1
  GreaterThanOrEqual1/1 -> Logical Operator/2
  Bus Selector/2 -> GreaterThanOrEqual1/1  "<MaxAzimuth>"
  In2/1 -> Abs/1
  Abs/1 -> GreaterThanOrEqual1/2

== system FusionMODEL_version4/OBJECT_TRACKER_SENSOR_FUSION/SENSOR_LAYOUT_AND_CHRACTERIZATION/PRE_COMPUTE_SENSOR_FOV_GRID/COMPUTE_RADAR_SNSR_GRID/ComputeCoverageANDConfidence/Compute_Cell_X_and_Y_index/Compute_FOV_Overlap_with_Cell_and_Region_Confidence/If Action Subsystem/Compute_Range_Azimuth ==
  x : Inport
  y : Inport  Port=2
  Add : Sum
  Atan : Trigonometry  Operator=atan
  Divide : Product  Inputs=*/
  Radians to Degrees : simulink_extras/Transformations/Radians to Degrees
  Sqrt : Sqrt  SaturateOnIntegerOverflow=on
  Square : Math  Operator=square  SaturateOnIntegerOverflow=on
  Square1 : Math  Operator=square  SaturateOnIntegerOverflow=on
  Range : Outport
  Azimuth : Outport  Port=2
  wires:
  Square/1 -> Add/1
  Square1/1 -> Add/2
  Add/1 -> Sqrt/1
  Atan/1 -> Radians to Degrees/1
  Sqrt/1 -> Range/1
  Radians to Degrees/1 -> Azimuth/1
  Divide/1 -> Atan/1
  y/1 -> Square1/1, Divide/1
  x/1 -> Square/1, Divide/2
